simulink model "full_bridge_Rectifier_using_Transformer"  (R2018b)
settings: Solver=VariableStepAuto  StartTime=0.0  StopTime=0.1  RelTol=1e-3
libraries: powerlib x12
settings Model: Creator=verma  LastModifiedBy=verma

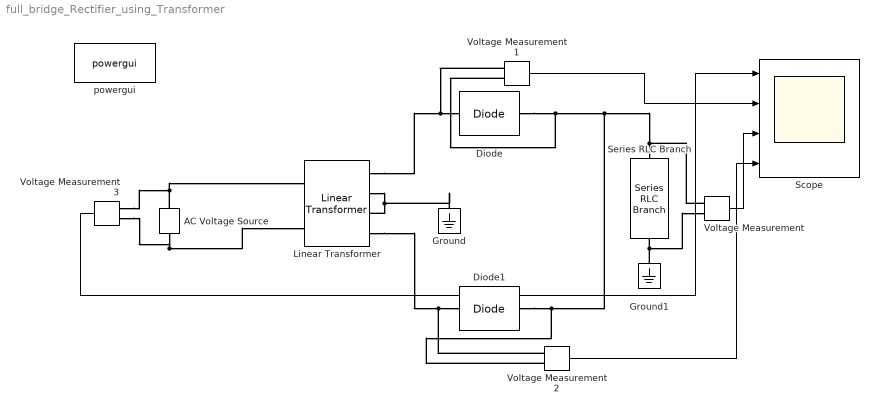
== system full_bridge_Rectifier_using_Transformer ==
  AC Voltage Source : powerlib/Electrical Sources/AC Voltage Source  Amplitude=30  Phase=0  Frequency=50  SampleTime=0  Measurements=None  BusType=swing  Pref=10e3  Qref=0  Qmin=-inf  Qmax=+inf
  Diode : powerlib/Power Electronics/Diode  Ron=0.0001  Lon=0  Vf=0.8  IC=0  UseSnubber=0  Rs=500  Cs=250e-9  Measurements=off
  Diode1 : powerlib/Power Electronics/Diode  Ron=0.0001  Lon=0  Vf=0.8  IC=0  UseSnubber=0  Rs=500  Cs=250e-9  Measurements=off
  Ground : powerlib/Elements/Ground  LConnTagsString=a
  Ground1 : powerlib/Elements/Ground  LConnTagsString=a
  Linear Transformer : powerlib/Elements/Linear Transformer  UNITS=pu  NominalPower=[ 250e6 60 ]  winding1="[ 14.14  0.000  0.00 ]"  winding2="[ 14.14  0.000  0.00  ]"  ThreeWindings=on  winding3="[ 14.14  0.000  0.00 ]"  RmLm=[inf inf]  Measurements=None  DataType=off
  Scope : Scope  NumInputPorts=4
  Series RLC Branch : powerlib/Elements/Series RLC Branch  LConnTagsString=__new0  RConnTagsString=__new0  BranchType=R  Resistance=500  Inductance=1e-3  SetiL0=off  InitialCurrent=0  Capacitance=1e-6  Setx0=off  InitialVoltage=0  Measurements=None
  Voltage Measurement{,1..3} (4 alike) : powerlib/Measurements/Voltage Measurement  PhasorSimulation=off  OutputType=Complex  PSBequivalent=0
  powergui : powerlib/powergui  Priority=1  SimulationMode=Continuous  SampleTime=50e-6  frequency=60  Iterations=50  frequencyindice=50  Pbase=100e6  ErrMax=1e-4  UnitsV=kV  UnitsW=MW  buscounter=0  FunctionMessages=off  echomessages=off  EnableUseOfTLC=off  CurrentSourceSwitches=off  DisableSnubberDevices=off  DisableRonSwitches=off  DisableVfSwitches=off  DisplayEquations=off  SolverType=Tustin/Backward Euler (TBE)  Interpol=off  ExternalGateDelay=off  methode=off  Ts=100  x0status=blocks  SPID=on  SwTol=0  HookPort=off  RestoreLinks=warning  ResistiveCurrentMeasurement=off  Frange=[0:2:500]  Ylog=off  Xlog=on  ShowGrid=off  save=off  variable=ZData  structure=0  ZoomFFT=off  StartTime=0.0  cycles=1  DisplayStyle=1  fundamental=60  FreqAxis=off  MaxFrequency=1000  frequencyindicesteady=1  RmsSteady=1  display=off
  wires:
  Voltage Measurement/1 -> Scope/3
  Voltage Measurement2/1 -> Scope/4
  Voltage Measurement1/1 -> Scope/2
  Voltage Measurement3/1 -> Scope/1
  connections:
  Linear Transformer/RConn1 -- Voltage Measurement1/LConn1 -- Diode/LConn1
  Linear Transformer/RConn4 -- Voltage Measurement2/LConn1 -- Diode1/LConn1
  AC Voltage Source/RConn1 -- Voltage Measurement3/LConn1 -- Linear Transformer/LConn1
  AC Voltage Source/LConn1 -- Voltage Measurement3/LConn2 -- Linear Transformer/LConn2
  Linear Transformer/RConn2 -- Ground/LConn1 -- Linear Transformer/RConn3
  Diode/RConn1 -- Voltage Measurement1/LConn2 -- Voltage Measurement2/LConn2 -- Diode1/RConn1 -- Voltage Measurement/LConn1 -- Series RLC Branch/LConn1
  Ground1/LConn1 -- Voltage Measurement/LConn2 -- Series RLC Branch/RConn1
